simulink model "hangji_source"  (R2020b)
settings: Solver=FixedStepAuto  StartTime=0.0  StopTime=100  FixedStep=0.01  RelTol=1e-3
settings Model: Creator=彭美祥  LastModifiedBy=彭美祥

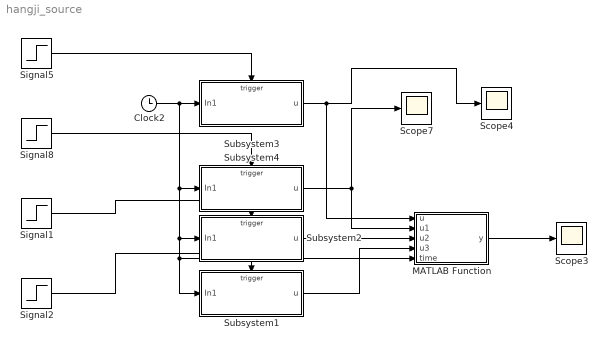
== system hangji_source ==
  Clock2 : Clock
  MATLAB Function : MATLAB Function  TreatAsAtomicUnit=on
  Scope3 : Scope
  Scope4 : Scope
  Scope7 : Scope
  Signal1 : Step  Time=30  SampleTime=0
  Signal2 : Step  Time=45  SampleTime=0
  Signal5 : Step  Time=2  SampleTime=0
  Signal8 : Step  Time=20  SampleTime=0
  Subsystem1 : Subsystem
  Subsystem2 : Subsystem
  Subsystem3 : Subsystem
  Subsystem4 : Subsystem
  wires:
  Signal5/1 -> Subsystem3/Trigger
  Signal8/1 -> Subsystem4/Trigger
  MATLAB Function/1(y) -> Scope3/1
  Subsystem3/1(u) -> MATLAB Function/1(u), Scope4/1
  Subsystem4/1(u) -> MATLAB Function/2(u1), Scope7/1
  Subsystem2/1(u) -> MATLAB Function/3(u2)
  Signal1/1 -> Subsystem2/Trigger
  Clock2/1 -> Subsystem2/1(In1), Subsystem1/1(In1), MATLAB Function/5(time), Subsystem4/1(In1), Subsystem3/1(In1)
  Subsystem1/1(u) -> MATLAB Function/4(u3)
  Signal2/1 -> Subsystem1/Trigger

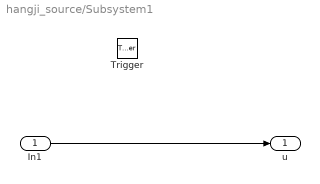
== system hangji_source/Subsystem1 ==
  In1 : Inport
  Trigger : TriggerPort  VariantControl=Variant  PortDimensions=1
  u : Outport
  wires:
  In1/1 -> u/1

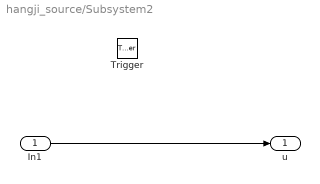
== system hangji_source/Subsystem2 ==
  In1 : Inport
  Trigger : TriggerPort  VariantControl=Variant  PortDimensions=1
  u : Outport
  wires:
  In1/1 -> u/1

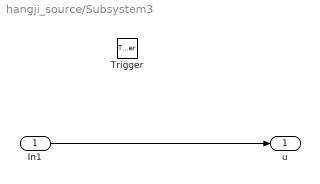
== system hangji_source/Subsystem3 ==
  In1 : Inport
  Trigger : TriggerPort  VariantControl=Variant  PortDimensions=1
  u : Outport
  wires:
  In1/1 -> u/1

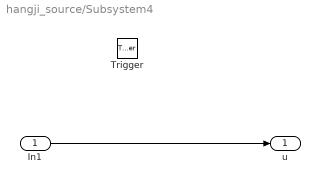
== system hangji_source/Subsystem4 ==
  In1 : Inport
  Trigger : TriggerPort  VariantControl=Variant  PortDimensions=1
  u : Outport
  wires:
  In1/1 -> u/1

== matlab function hangji_source/MATLAB Function ==
  data: u input; u1 input; u2 input; u3 input; y output; time input
function y = fcn(u,u1,u2,u3,time)
if u<=0
    y = -600;
else
    if time < u+2
        y = -600;
    else
        y = (time-u-2)*(-290+600)/(50-3)-600; 
    end
    if u1 <= 0
    else
        if time > u1+2
            y = (u1+2-u-2)*(-290+600)/(50-3)-600;
        end
    end
    if u2 <= 0
    else
        if time > u2+2
            y_ini = (u1+2-u-2)*(-290+600)/(50-3)-600;
            y = (time-u2-2)*(-290+600)/(50-3)+y_ini;
        end
    end
    if u3 <=0
    else
        if time > u3+2
            y1_ini = (u1+2-u-2)*(-290+600)/(50-3)-600;
            y2_ini = y1_ini;
            y3_ini = (u3+2-u2-2)*(-290+600)/(50-3)+y2_ini;
            y = (time-u3-2)*290/(64-50)+y3_ini;
        end
    end 
    if y >= 0
        y = 0;
    end
end

end
% function y = fcn(u,u1,u2,u3,time)
% if u <= 0 
%     y = -600;
% else
%     if time < (u+2)
%         y = -600;
%     elseif time <= (u+2+47)
%         if u1 > 0 
%             if time < u1 + 2       
%                 y = (time-u-2)*(-290+600)/(50-3)+y_ini;
%             else
%                 y_ini = (u1+2-u-2)*(-290+600)/(50-3)-600;
%                 y = (time-u1-2)*290/(64-50) + y_ini;            
%             end
%         elseif u2>0
%             y_ini = (u2-u-2)*(-290+600)/(50-3)-600;
%             y = y_ini;
%             if u3>0
%                 y = (time+2-u3-2)*(-290+600)/(50-3)+ y_ini; 
%             end
%         else
%             y = (time-u-2)*(-290+600)/(50-3)-600; 
%         end
%     elseif time <= (u+2+47+14)
%         if u1 > 0
%             y_ini = (u1+2-u-2)*(-290+600)/(50-3)-600;
%             y = (time-u1-2)*290/(64-50) + y_ini;
%         else
%             y = (time-u-2-47)*290/(64-50)-290;
%         end
%     else
%         y = 0;
%     end
%     if y >= 0
%         y = 0;
%     end
% end
